simulink model "disctrete_PID_dist_delay"  (R2017a)
settings: Solver=VariableStepAuto  StartTime=0.0  StopTime=1  RelTol=1e-3
values from neighbouring files (symbols this model uses):
  h2 = 0.0015    [q3.m]    (also in q3_reduced.m = 0.003)
undefined symbols (not defined in the file or in its folder): A2, A_dr, B2, B_dr, C2, C_dr, D2, D_dr
settings Model: Creator=Aleksandra  LastModifiedBy=Aleksandra

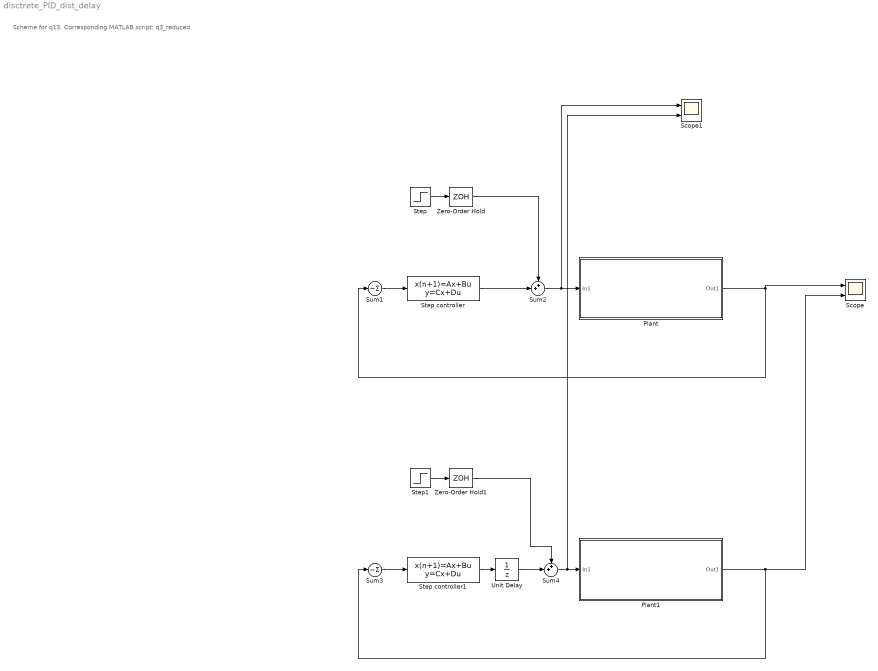
== system disctrete_PID_dist_delay ==
  note: Scheme for q13.
      | Corresponding MATLAB script: q3_reduced
  Plant : Subsystem
  Plant1 : Subsystem
  Scope : Scope  NumInputPorts=2
  Scope1 : Scope  NumInputPorts=2
  Step : Step  Time=0  SampleTime=0
  Step controller : DiscreteStateSpace  A=A_dr  B=B_dr  C=C_dr  D=D_dr  SampleTime=h2
  Step controller1 : DiscreteStateSpace  A=A_dr  B=B_dr  C=C_dr  D=D_dr  SampleTime=h2
  Step1 : Step  Time=0  SampleTime=0
  Sum1 : Sum  Inputs=-
  Sum2 : Sum  Inputs=++|
  Sum3 : Sum  Inputs=-
  Sum4 : Sum  Inputs=++|
  Unit Delay : UnitDelay  SampleTime=-1
  Zero-Order Hold : ZeroOrderHold  SampleTime=h2
  Zero-Order Hold1 : ZeroOrderHold  SampleTime=h2
  wires:
  Zero-Order Hold/1 -> Sum2/1
  Step/1 -> Zero-Order Hold/1
  Plant/1(Out1) -> Sum1/1, Scope/1
  Step controller/1 -> Sum2/2
  Sum2/1 -> Scope1/1, Plant/1(In1)
  Sum1/1 -> Step controller/1
  Sum3/1 -> Step controller1/1
  Step1/1 -> Zero-Order Hold1/1
  Sum4/1 -> Scope1/2, Plant1/1(In1)
  Zero-Order Hold1/1 -> Sum4/1
  Step controller1/1 -> Unit Delay/1
  Plant1/1(Out1) -> Scope/2, Sum3/1
  Unit Delay/1 -> Sum4/2

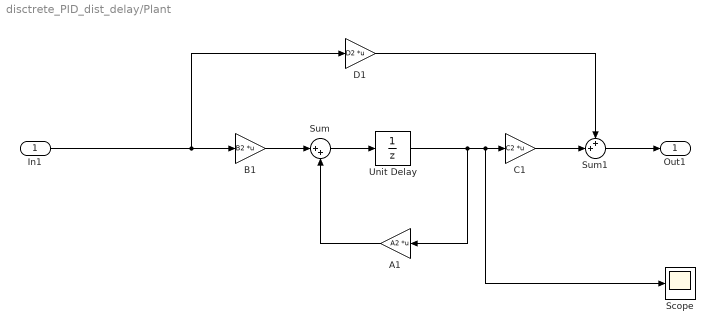
== system disctrete_PID_dist_delay/Plant ==
  In1 : Inport
  A1 : Gain  Gain=A2  Multiplication=Matrix(K*u)
  B1 : Gain  Gain=B2  Multiplication=Matrix(K*u)
  C1 : Gain  Gain=C2  Multiplication=Matrix(K*u)
  D1 : Gain  Gain=D2  Multiplication=Matrix(K*u)
  Scope : Scope
  Sum : Sum  Inputs=|++
  Sum1 : Sum  Inputs=++|
  Unit Delay : UnitDelay  SampleTime=-1
  Out1 : Outport
  wires:
  In1/1 -> D1/1, B1/1
  A1/1 -> Sum/2
  Sum/1 -> Unit Delay/1
  C1/1 -> Sum1/2
  Sum1/1 -> Out1/1
  D1/1 -> Sum1/1
  B1/1 -> Sum/1
  Unit Delay/1 -> A1/1, Scope/1, C1/1

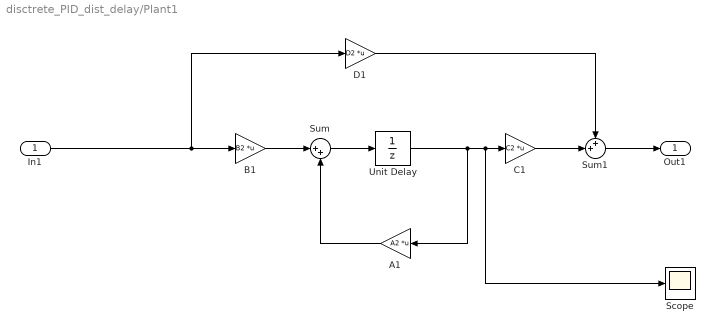
== system disctrete_PID_dist_delay/Plant1 ==
  In1 : Inport
  A1 : Gain  Gain=A2  Multiplication=Matrix(K*u)
  B1 : Gain  Gain=B2  Multiplication=Matrix(K*u)
  C1 : Gain  Gain=C2  Multiplication=Matrix(K*u)
  D1 : Gain  Gain=D2  Multiplication=Matrix(K*u)
  Scope : Scope
  Sum : Sum  Inputs=|++
  Sum1 : Sum  Inputs=++|
  Unit Delay : UnitDelay  SampleTime=-1
  Out1 : Outport
  wires:
  In1/1 -> D1/1, B1/1
  A1/1 -> Sum/2
  Sum/1 -> Unit Delay/1
  C1/1 -> Sum1/2
  Sum1/1 -> Out1/1
  D1/1 -> Sum1/1
  B1/1 -> Sum/1
  Unit Delay/1 -> A1/1, Scope/1, C1/1
